simulink model "lead_p1"  (R2017a)
settings: Solver=ode45  StartTime=0.0  StopTime=1  MaxStep=0.001  RelTol=1e-3
values from neighbouring files (symbols this model uses):
  K = 18    [lab6.m]    (also in prelab6.m)
  Ka = 2.4    [lab6.m]
  Kc = 3    [lab6.m]
  Kp = 10/(2*pi)    (= 1.59154943092)    [lab6.m]
  Tm = 2/10    (= 0.2)    [lab6.m]
  Tp = 1/200    (= 0.005)    [lab6.m]
  Tz = 1/10    (= 0.1)    [lab6.m]
  VS = .5    (= 0.5)    [lab6.m]
settings Model: Creator=vjdixit2  LastModifiedBy=vjdixit2

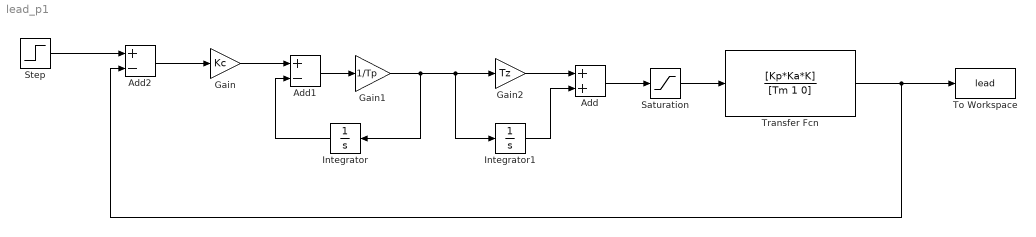
== system lead_p1 ==
  Add : Sum
  Add1 : Sum  Inputs=+-
  Add2 : Sum  Inputs=+-
  Gain : Gain  Gain=Kc
  Gain1 : Gain  Gain=1/Tp
  Gain2 : Gain  Gain=Tz
  Integrator : Integrator
  Integrator1 : Integrator
  Saturation : Saturate  UpperLimit=inf  LowerLimit=-inf
  Step : Step  Time=0  After=VS  SampleTime=0
  To Workspace : ToWorkspace  VariableName=lead  SampleTime=-1
  Transfer Fcn : TransferFcn  Numerator=[Kp*Ka*K]  Denominator=[Tm 1 0]
  wires:
  Add/1 -> Saturation/1
  Gain2/1 -> Add/1
  Integrator1/1 -> Add/2
  Add1/1 -> Gain1/1
  Integrator/1 -> Add1/2
  Gain1/1 -> Integrator1/1, Gain2/1, Integrator/1
  Gain/1 -> Add1/1
  Saturation/1 -> Transfer Fcn/1
  Transfer Fcn/1 -> Add2/2, To Workspace/1
  Step/1 -> Add2/1
  Add2/1 -> Gain/1
